simulink model "Dynamics_v2_temp"  (R2021b)
settings: Solver=VariableStepAuto  StartTime=0.0  StopTime=10.0  RelTol=1e-3
InitFcn:
  | % ************** Initiate forces
  | % f0=[0;0;0;0;0;0];
  | % f0=[0;0;0;0;0;0;0];
  | f_0=[0;0;0];
  | f_m=[0;0];
  | f_e=[0;0;0;0;0;0];
  | % ************** Initiate states
  | q_m=[0;0];
  | q_dot_m=[0;0];
  | P=[0;0;0];
  | V_I0=[0;0;0];
  | % ************** Load main
  | %run(Main.m)
values from neighbouring files (symbols this model uses):
  diag_M = diagonalize(M_frak0, M_frak)    [Create_Robot.m]    (also in Main.m; diagonalize.m = zeros(6*(n+1),6*(n+1)); test_C_Main.m)
  iota0 = [1 0 0; 0 1 0;zeros(3,3);0 0 1]    [Create_Robot.m]    (also in Main.m = eye(6,6); test_C_Main.m)
  M_curly = zeros(n,6,6)    [M_curly.m]
  mu = zeros(6,1)'    [Create_Robot.m]    (also in Main.m; test_C_Main.m)
  Xi_m_matrix = zeros(6*n,n)    [Create_Robot.m]    (also in Main.m; test_C_Main.m)
undefined symbols (not defined in the file or in its folder): Ad_gm_inv, g_bar, M_curly0, Xi_m
(part 1 of 2)
settings Model: Creator=Bmmog  LastModifiedBy=Bmmog

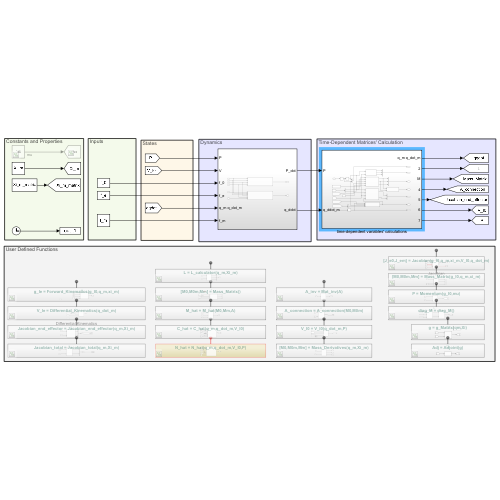
[thumbnail: Simulink's stored preview of the top-level diagram]
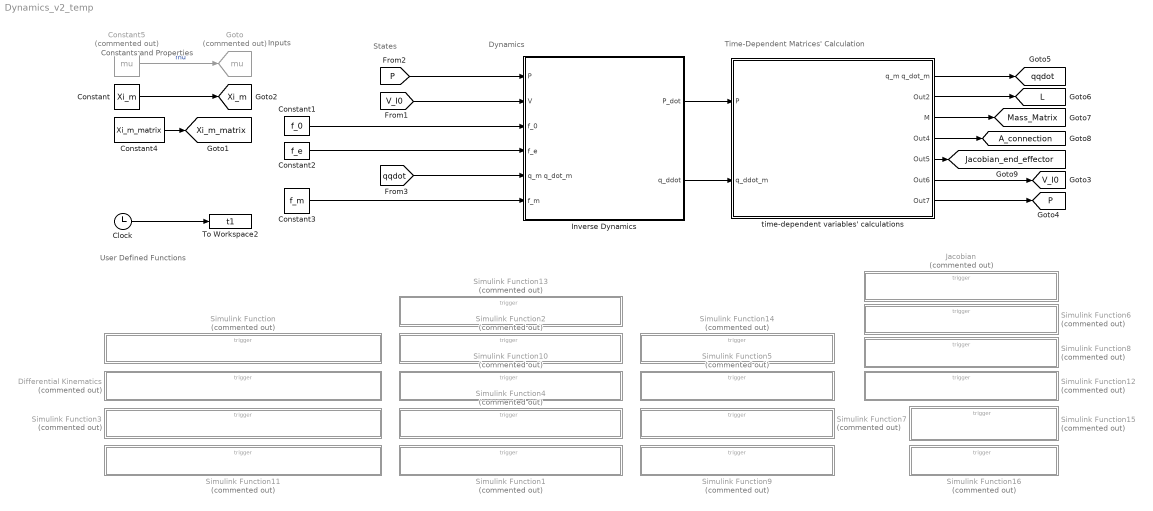
== system Dynamics_v2_temp ==
  note: Time-Dependent Matrices' Calculation
  note: States
  note: Inputs
  note: User Defined Functions
  note: Dynamics
  note: Constants and Properties
  Clock : Clock
  Constant : Constant  Value=Xi_m  VectorParams1D=off
  Constant1 : Constant  Value=f_0  VectorParams1D=off
  Constant2 : Constant  Value=f_e  VectorParams1D=off
  Constant3 : Constant  Value=f_m  VectorParams1D=off
  Constant4 : Constant  Value=Xi_m_matrix  VectorParams1D=off
  Constant5 : Constant  Commented=on  Value=mu
  Differential Kinematics : Subsystem  Commented=on  TreatAsAtomicUnit=on
  Goto : Goto  Commented=on  GotoTag=mu  TagVisibility=global
  Inverse Dynamics : Subsystem
  Jacobian : Subsystem  Commented=on  TreatAsAtomicUnit=on
  Simulink Function : Subsystem  Commented=on  TreatAsAtomicUnit=on
  Simulink Function1 : Subsystem  Commented=on  TreatAsAtomicUnit=on
  Simulink Function10 : Subsystem  Commented=on  TreatAsAtomicUnit=on
  Simulink Function11 : Subsystem  Commented=on  TreatAsAtomicUnit=on
  Simulink Function12 : Subsystem  Commented=on  TreatAsAtomicUnit=on
  Simulink Function13 : Subsystem  Commented=on  TreatAsAtomicUnit=on
  Simulink Function14 : Subsystem  Commented=on  TreatAsAtomicUnit=on
  Simulink Function15 : Subsystem  Commented=on  TreatAsAtomicUnit=on
  Simulink Function16 : Subsystem  Commented=on  TreatAsAtomicUnit=on
  Simulink Function2 : Subsystem  Commented=on  TreatAsAtomicUnit=on
  Simulink Function3 : Subsystem  Commented=on  TreatAsAtomicUnit=on
  Simulink Function4 : Subsystem  Commented=on  TreatAsAtomicUnit=on
  Simulink Function5 : Subsystem  Commented=on  TreatAsAtomicUnit=on
  Simulink Function6 : Subsystem  Commented=on  TreatAsAtomicUnit=on
  Simulink Function7 : Subsystem  Commented=on  TreatAsAtomicUnit=on
  Simulink Function8 : Subsystem  Commented=on  TreatAsAtomicUnit=on
  Simulink Function9 : Subsystem  Commented=on  TreatAsAtomicUnit=on
  To Workspace2 : ToWorkspace  VariableName=t1  SampleTime=-1
  time-dependent variables' calculations : Subsystem
  tag scope: A_connection=global, Jacobian_end_effector=global, L=global, Mass_Matrix=global, P=global, V_I0=global, Xi_m=global, Xi_m_matrix=global, qqdot=global
  wires:
  Constant5/1 -> Goto/1  "mu"
  Clock/1 -> To Workspace2/1
  Constant/1 -> [Xi_m]
  Constant4/1 -> [Xi_m_matrix]
  Constant1/1 -> Inverse Dynamics/3(f_0)
  Constant2/1 -> Inverse Dynamics/4(f_e)
  Constant3/1 -> Inverse Dynamics/6(f_m)
  [P] -> Inverse Dynamics/1(P)
  [V_I0] -> Inverse Dynamics/2(V)
  [qqdot] -> Inverse Dynamics/5(q_m q_dot_m)
  time-dependent variables' calculations/7(Out7) -> [P]
  time-dependent variables' calculations/6(Out6) -> [V_I0]
  time-dependent variables' calculations/5(Out5) -> [Jacobian_end_effector]
  time-dependent variables' calculations/4(Out4) -> [A_connection]
  time-dependent variables' calculations/3(M) -> [Mass_Matrix]
  time-dependent variables' calculations/2(Out2) -> [L]
  time-dependent variables' calculations/1(q_m q_dot_m) -> [qqdot]
  Inverse Dynamics/1(P_dot) -> time-dependent variables' calculations/1(P)
  Inverse Dynamics/2(q_ddot) -> time-dependent variables' calculations/2(q_ddot_m)

== system Dynamics_v2_temp/Differential Kinematics ==
  Differential_Kinematics : TriggerPort  TriggerType=function-call  IsSimulinkFunction=on  FunctionName=Differential_Kinematics  FunctionVisibility=scoped  VariantControl=(inherit)
  Demux : Demux  Outputs=2
  From2 : From  Commented=on  GotoTag=A_connection  TagVisibility=global
  MATLAB Function : MATLAB Function  TreatAsAtomicUnit=on
  q_dot_m : ArgIn  DisableCoverage=on  ArgumentName=q_dot_m
  V_Ie : ArgOut  DisableCoverage=on  ArgumentName=V_Ie
  wires:
  MATLAB Function/1(V_Ie) -> V_Ie/1
  q_dot_m/1 -> MATLAB Function/1(q_dot_m)
  Demux/1 -> MATLAB Function/2(J_e0)
  Demux/2 -> MATLAB Function/3(J_em)
  [Jacobian_end_effector] -> Demux/1
  [V_I0] -> MATLAB Function/4(V_I0)

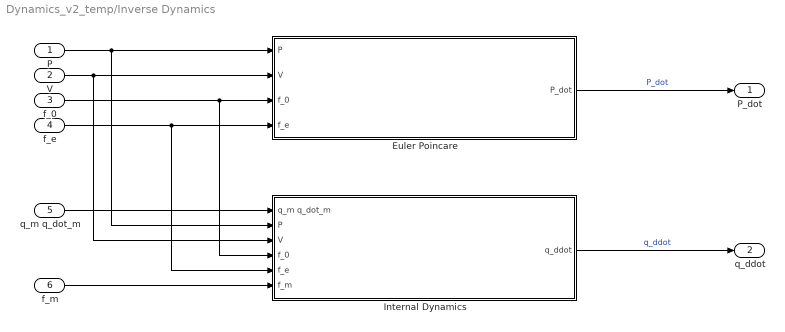
== system Dynamics_v2_temp/Inverse Dynamics ==
  P : Inport
  V : Inport  Port=2
  f_0 : Inport  Port=3
  f_e : Inport  Port=4
  q_m q_dot_m : Inport  Port=5
  f_m : Inport  Port=6
  Euler Poincare : Subsystem
  Internal Dynamics : Subsystem
  P_dot : Outport
  q_ddot : Outport  Port=2
  wires:
  f_0/1 -> Internal Dynamics/4(f_0), Euler Poincare/3(f_0)
  f_e/1 -> Internal Dynamics/5(f_e), Euler Poincare/4(f_e)
  f_m/1 -> Internal Dynamics/6(f_m)
  Internal Dynamics/1(q_ddot) -> q_ddot/1  "q_ddot"
  Euler Poincare/1(P_dot) -> P_dot/1  "P_dot"
  q_m q_dot_m/1 -> Internal Dynamics/1(q_m q_dot_m)
  P/1 -> Internal Dynamics/2(P), Euler Poincare/1(P)
  V/1 -> Internal Dynamics/3(V), Euler Poincare/2(V)

== system Dynamics_v2_temp/Jacobian ==
  Jacobian : TriggerPort  TriggerType=function-call  IsSimulinkFunction=on  FunctionName=Jacobian  FunctionVisibility=scoped  VariantControl=(inherit)
  MATLAB Function : MATLAB Function  TreatAsAtomicUnit=on
  g_I0 : ArgIn  DisableCoverage=on  ArgumentName=g_I0
  q_m : ArgIn  DisableCoverage=on  Port=2  ArgumentName=q_m
  xi_m : ArgIn  DisableCoverage=on  Port=3  ArgumentName=xi_m
  V_I0 : ArgIn  DisableCoverage=on  Port=4  ArgumentName=V_I0
  q_dot_m : ArgIn  DisableCoverage=on  Port=5  ArgumentName=q_dot_m
  J_e0 : ArgOut  DisableCoverage=on  ArgumentName=J_e0
  J_em : ArgOut  DisableCoverage=on  Port=2  ArgumentName=J_em
  wires:
  g_I0/1 -> MATLAB Function/1(robot)
  MATLAB Function/1(J) -> J_e0/1
  q_m/1 -> MATLAB Function/2(q)
  xi_m/1 -> ?
  q_dot_m/1 -> ?
  V_I0/1 -> ?
  ? -> J_em/1

== system Dynamics_v2_temp/Simulink Function ==
  Forward_Kinematics : TriggerPort  TriggerType=function-call  IsSimulinkFunction=on  FunctionName=Forward_Kinematics  FunctionVisibility=scoped  VariantControl=(inherit)
  Constant : Constant  Value=g_bar
  From : From  Commented=on  GotoTag=g_bar
  MATLAB Function : MATLAB Function  TreatAsAtomicUnit=on
  g_I0 : ArgIn  DisableCoverage=on  ArgumentName=g_I0
  q_m : ArgIn  DisableCoverage=on  Port=2  ArgumentName=q_m
  xi_m : ArgIn  DisableCoverage=on  Port=3  ArgumentName=xi_m
  g_Ie : ArgOut  DisableCoverage=on  ArgumentName=g_Ie
  wires:
  g_I0/1 -> MATLAB Function/1(g_I0)
  MATLAB Function/1(g_Ie) -> g_Ie/1
  q_m/1 -> MATLAB Function/2(q_m)
  xi_m/1 -> MATLAB Function/3(Xi_m)
  Constant/1 -> MATLAB Function/4(g_bar)

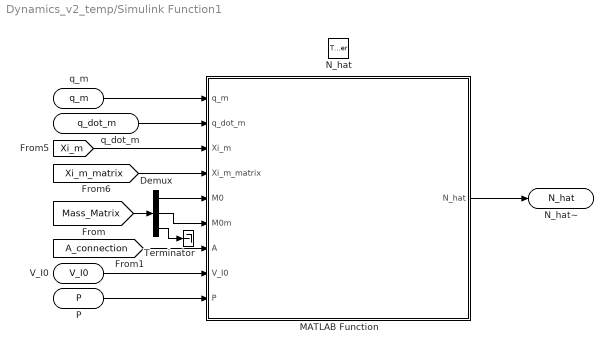
== system Dynamics_v2_temp/Simulink Function1 ==
  N_hat : TriggerPort  TriggerType=function-call  IsSimulinkFunction=on  FunctionName=N_hat  FunctionVisibility=scoped  VariantControl=(inherit)
  Demux : Demux  Outputs=3
  MATLAB Function : MATLAB Function  TreatAsAtomicUnit=on
  Terminator : Terminator
  q_m : ArgIn  DisableCoverage=on  ArgumentName=q_m
  q_dot_m : ArgIn  DisableCoverage=on  Port=2  ArgumentName=q_dot_m
  V_I0 : ArgIn  DisableCoverage=on  Port=3  ArgumentName=V_I0
  P : ArgIn  DisableCoverage=on  Port=4  ArgumentName=P
  N_hat~ : ArgOut  DisableCoverage=on  ArgumentName=N_hat
  wires:
  MATLAB Function/1(N_hat) -> N_hat~/1
  q_m/1 -> MATLAB Function/1(q_m)
  [Xi_m] -> MATLAB Function/3(Xi_m)
  q_dot_m/1 -> MATLAB Function/2(q_dot_m)
  [Xi_m_matrix] -> MATLAB Function/4(Xi_m_matrix)
  [Mass_Matrix] -> Demux/1
  Demux/1 -> MATLAB Function/5(M0)
  Demux/2 -> MATLAB Function/6(M0m)
  Demux/3 -> Terminator/1
  [A_connection] -> MATLAB Function/7(A)
  V_I0/1 -> MATLAB Function/8(V_I0)
  P/1 -> MATLAB Function/9(P)

== system Dynamics_v2_temp/Simulink Function10 ==
  M_hat : TriggerPort  TriggerType=function-call  IsSimulinkFunction=on  FunctionName=M_hat  FunctionVisibility=scoped  VariantControl=(inherit)
  MATLAB Function : MATLAB Function  TreatAsAtomicUnit=on
  M0 : ArgIn  DisableCoverage=on  ArgumentName=M0
  M0m : ArgIn  DisableCoverage=on  Port=2  ArgumentName=Mm
  A : ArgIn  DisableCoverage=on  Port=3  ArgumentName=A
  M_hat~ : ArgOut  DisableCoverage=on  ArgumentName=M_hat
  wires:
  MATLAB Function/1(M_hat) -> M_hat~/1
  M0m/1 -> MATLAB Function/2(Mm)
  A/1 -> MATLAB Function/3(A)
  M0/1 -> MATLAB Function/1(M0)

== system Dynamics_v2_temp/Simulink Function11 ==
  Jacobian_total : TriggerPort  TriggerType=function-call  IsSimulinkFunction=on  FunctionName=Jacobian_total  FunctionVisibility=scoped  VariantControl=(inherit)
  MATLAB Function : MATLAB Function  TreatAsAtomicUnit=on
  Mux : Mux  Inputs=2
  q_m : ArgIn  DisableCoverage=on  ArgumentName=q_m
  Xi_m : ArgIn  DisableCoverage=on  Port=2  ArgumentName=Xi_m
  Jacobian_total~ : ArgOut  DisableCoverage=on  ArgumentName=Jacobian_total
  wires:
  MATLAB Function/1(J_e0) -> Mux/1
  q_m/1 -> MATLAB Function/1(q_m)
  Xi_m/1 -> MATLAB Function/2(Xi_m)
  MATLAB Function/2(J_em) -> Mux/2
  Mux/1 -> Jacobian_total~/1

== system Dynamics_v2_temp/Simulink Function12 ==
  diag_M : TriggerPort  TriggerType=function-call  IsSimulinkFunction=on  FunctionName=diag_M  FunctionVisibility=scoped  VariantControl=(inherit)
  Constant : Constant  Value=M_curly0
  Constant1 : Constant  Value=M_curly
  Constant2 : Constant  Value=Ad_gm_inv
  MATLAB Function : MATLAB Function  TreatAsAtomicUnit=on
  MATLAB Function1 : MATLAB Function  TreatAsAtomicUnit=on
  diag_M~ : ArgOut  DisableCoverage=on  ArgumentName=diag_M
  wires:
  MATLAB Function/2(M_frak) -> MATLAB Function1/2(M_frak)
  MATLAB Function1/1(diag_M) -> diag_M~/1
  Constant/1 -> MATLAB Function/1(M_curly0)
  Constant1/1 -> MATLAB Function/2(M_curly)
  Constant2/1 -> MATLAB Function/3(Ad_gm_inv)
  MATLAB Function/1(M_frak0) -> MATLAB Function1/1(M_frak0)

== system Dynamics_v2_temp/Simulink Function13 ==
  L_calculator : TriggerPort  TriggerType=function-call  IsSimulinkFunction=on  FunctionName=L_calculator  FunctionVisibility=scoped  VariantControl=(inherit)
  " " : MATLAB Function  TreatAsAtomicUnit=on
  Mux : Mux  Inputs=3
  q_m : ArgIn  DisableCoverage=on  ArgumentName=q_m
  Xi_m : ArgIn  DisableCoverage=on  Port=2  ArgumentName=Xi_m
  L : ArgOut  DisableCoverage=on  ArgumentName=L
  wires:
  " "/1(L0) -> Mux/1
  Xi_m/1 -> " "/2(Xi_m)
  " "/2(Lm0) -> Mux/2
  Mux/1 -> L/1
  " "/3(Lm) -> Mux/3
  q_m/1 -> " "/1(q_m)

== system Dynamics_v2_temp/Simulink Function14 ==
  Mat_inv : TriggerPort  TriggerType=function-call  IsSimulinkFunction=on  FunctionName=Mat_inv  FunctionVisibility=scoped  VariantControl=(inherit)
  MATLAB Function1 : MATLAB Function  TreatAsAtomicUnit=on
  A : ArgIn  DisableCoverage=on  ArgumentName=A
  A_inv : ArgOut  DisableCoverage=on  ArgumentName=A_inv
  wires:
  A/1 -> MATLAB Function1/1(A)
  MATLAB Function1/1(A_inv) -> A_inv/1

== system Dynamics_v2_temp/Simulink Function15 ==
  g_Matrix : TriggerPort  TriggerType=function-call  IsSimulinkFunction=on  FunctionName=g_Matrix  FunctionVisibility=scoped  VariantControl=(inherit)
  MATLAB Function : MATLAB Function  Commented=on  TreatAsAtomicUnit=on
  MATLAB Function1 : MATLAB Function  TreatAsAtomicUnit=on
  qm : ArgIn  DisableCoverage=on  ArgumentName=qm
  Xi : ArgIn  DisableCoverage=on  Port=2  ArgumentName=Xi
  g : ArgOut  DisableCoverage=on  ArgumentName=g
  wires:
  qm/1 -> MATLAB Function1/2(qm)
  Xi/1 -> MATLAB Function1/1(xi)
  MATLAB Function1/1(g) -> g/1

== system Dynamics_v2_temp/Simulink Function16 ==
  Adjoint : TriggerPort  TriggerType=function-call  IsSimulinkFunction=on  FunctionName=Adjoint  FunctionVisibility=scoped  VariantControl=(inherit)
  MATLAB Function : MATLAB Function  TreatAsAtomicUnit=on
  u : ArgIn  DisableCoverage=on  ArgumentName=g
  y : ArgOut  DisableCoverage=on  ArgumentName=Adj
  wires:
  u/1 -> MATLAB Function/1(g)
  MATLAB Function/1(Adj) -> y/1

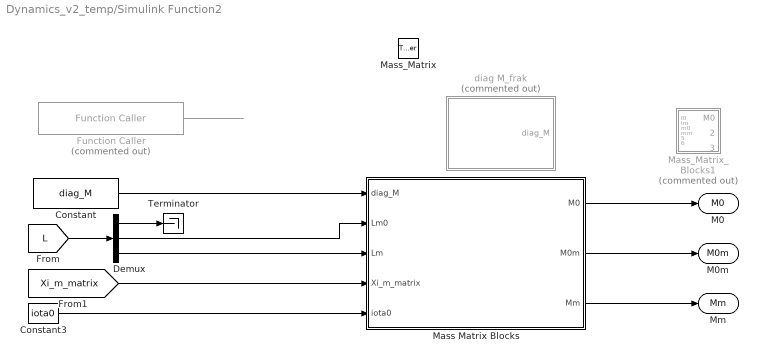
== system Dynamics_v2_temp/Simulink Function2 ==
  Mass_Matrix : TriggerPort  TriggerType=function-call  IsSimulinkFunction=on  FunctionName=Mass_Matrix  FunctionVisibility=scoped  VariantControl=(inherit)
  Constant : Constant  Value=diag_M  VectorParams1D=off
  Constant3 : Constant  Value=iota0  VectorParams1D=off
  Demux : Demux  Outputs=3
  Function Caller : FunctionCaller  Commented=on  FunctionPrototype=diag_M = diag_M()  InputArgumentSpecifications=<Enter example>  OutputArgumentSpecifications=<Enter example>
  Mass Matrix Blocks : Subsystem
  Mass_Matrix_Blocks1 : MATLAB Function  Commented=on  TreatAsAtomicUnit=on
  Terminator : Terminator
  diag M_frak : Subsystem  Commented=on
  M0 : ArgOut  DisableCoverage=on  ArgumentName=M0
  M0m : ArgOut  DisableCoverage=on  Port=2  ArgumentName=M0m
  Mm : ArgOut  DisableCoverage=on  Port=3  ArgumentName=Mm
  wires:
  [L] -> Demux/1
  Demux/1 -> Terminator/1
  Demux/2 -> Mass Matrix Blocks/2(Lm0)
  Demux/3 -> Mass Matrix Blocks/3(Lm)
  [Xi_m_matrix] -> Mass Matrix Blocks/4(Xi_m_matrix)
  Constant3/1 -> Mass Matrix Blocks/5(iota0)
  Mass Matrix Blocks/1(M0) -> M0/1
  Mass Matrix Blocks/2(M0m) -> M0m/1
  Mass Matrix Blocks/3(Mm) -> Mm/1
  Function Caller/1 -> ?
  Constant/1 -> Mass Matrix Blocks/1(diag_M)

== system Dynamics_v2_temp/Simulink Function3 ==
  Jacobian_end_effector : TriggerPort  TriggerType=function-call  IsSimulinkFunction=on  FunctionName=Jacobian_end_effector  FunctionVisibility=scoped  VariantControl=(inherit)
  MATLAB Function : MATLAB Function  TreatAsAtomicUnit=on
  Mux : Mux  Inputs=2
  q_m : ArgIn  DisableCoverage=on  ArgumentName=q_m
  Xi_m : ArgIn  DisableCoverage=on  Port=2  ArgumentName=Xi_m
  Jacobian_end_effector~ : ArgOut  DisableCoverage=on  ArgumentName=Jacobian_end_effector
  wires:
  MATLAB Function/1(J_e0) -> Mux/1
  q_m/1 -> MATLAB Function/1(q_m)
  Xi_m/1 -> MATLAB Function/2(Xi_m)
  MATLAB Function/2(J_em) -> Mux/2
  Mux/1 -> Jacobian_end_effector~/1

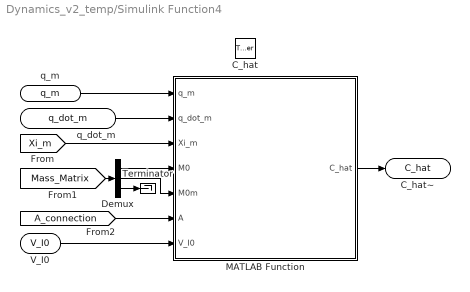
== system Dynamics_v2_temp/Simulink Function4 ==
  C_hat : TriggerPort  TriggerType=function-call  IsSimulinkFunction=on  FunctionName=C_hat  FunctionVisibility=scoped  VariantControl=(inherit)
  Demux : Demux  Outputs=3
  MATLAB Function : MATLAB Function  TreatAsAtomicUnit=on
  Terminator : Terminator
  q_m : ArgIn  DisableCoverage=on  ArgumentName=q_m
  q_dot_m : ArgIn  DisableCoverage=on  Port=2  ArgumentName=q_dot_m
  V_I0 : ArgIn  DisableCoverage=on  Port=3  ArgumentName=V_I0
  C_hat~ : ArgOut  DisableCoverage=on  ArgumentName=C_hat
  wires:
  [Mass_Matrix] -> Demux/1
  MATLAB Function/1(C_hat) -> C_hat~/1
  q_m/1 -> MATLAB Function/1(q_m)
  [Xi_m] -> MATLAB Function/3(Xi_m)
  q_dot_m/1 -> MATLAB Function/2(q_dot_m)
  [A_connection] -> MATLAB Function/6(A)
  Demux/3 -> Terminator/1
  Demux/1 -> MATLAB Function/4(M0)
  Demux/2 -> MATLAB Function/5(M0m)
  V_I0/1 -> MATLAB Function/7(V_I0)

== system Dynamics_v2_temp/Simulink Function5 ==
  A_connection : TriggerPort  TriggerType=function-call  IsSimulinkFunction=on  FunctionName=A_connection  FunctionVisibility=scoped  VariantControl=(inherit)
  MATLAB Function : MATLAB Function  TreatAsAtomicUnit=on
  M0 : ArgIn  DisableCoverage=on  ArgumentName=M0
  M0m : ArgIn  DisableCoverage=on  Port=2  ArgumentName=M0m
  A_connection~ : ArgOut  DisableCoverage=on  ArgumentName=A_connection
  wires:
  M0/1 -> MATLAB Function/1(M0)
  MATLAB Function/1(A) -> A_connection~/1
  M0m/1 -> MATLAB Function/2(M0m)

== system Dynamics_v2_temp/Simulink Function6 ==
  Mass_Matrix : TriggerPort  TriggerType=function-call  IsSimulinkFunction=on  FunctionName=Mass_Matrix  FunctionVisibility=scoped  VariantControl=(inherit)
  MATLAB Function : MATLAB Function  TreatAsAtomicUnit=on
  g_I0 : ArgIn  DisableCoverage=on  ArgumentName=g_I0
  q_m : ArgIn  DisableCoverage=on  Port=2  ArgumentName=q_m
  xi_m : ArgIn  DisableCoverage=on  Port=3  ArgumentName=xi_m
  M0 : ArgOut  DisableCoverage=on  ArgumentName=M0
  M0m : ArgOut  DisableCoverage=on  Port=2  ArgumentName=M0m
  Mm : ArgOut  DisableCoverage=on  Port=3  ArgumentName=Mm
  wires:
  g_I0/1 -> MATLAB Function/1(I0)
  MATLAB Function/1(M0) -> M0/1
  q_m/1 -> MATLAB Function/7(q_m)
  xi_m/1 -> MATLAB Function/8(Xi_m)
  MATLAB Function/2(M0m) -> M0m/1
  MATLAB Function/3(Mm) -> Mm/1

== system Dynamics_v2_temp/Simulink Function7 ==
  V_I0 : TriggerPort  TriggerType=function-call  IsSimulinkFunction=on  FunctionName=V_I0  FunctionVisibility=scoped  VariantControl=(inherit)
  Demux : Demux  Outputs=3
  MATLAB Function : MATLAB Function  TreatAsAtomicUnit=on
  Terminator : Terminator
  Terminator1 : Terminator
  q_dot_m : ArgIn  DisableCoverage=on  ArgumentName=q_dot_m
  P : ArgIn  DisableCoverage=on  Port=2  ArgumentName=P
  V_I0~ : ArgOut  DisableCoverage=on  ArgumentName=V_I0
  wires:
  Demux/1 -> MATLAB Function/4(M0)
  MATLAB Function/1(V_I0) -> V_I0~/1
  P/1 -> MATLAB Function/1(P)
  [Mass_Matrix] -> Demux/1
  Demux/2 -> Terminator/1
  Demux/3 -> Terminator1/1
  [A_connection] -> MATLAB Function/2(A_connection)
  q_dot_m/1 -> MATLAB Function/3(q_dot_m)

== system Dynamics_v2_temp/Simulink Function8 ==
  Momentum : TriggerPort  TriggerType=function-call  IsSimulinkFunction=on  FunctionName=Momentum  FunctionVisibility=scoped  VariantControl=(inherit)
  MATLAB Function : MATLAB Function  TreatAsAtomicUnit=on
  g_I0 : ArgIn  DisableCoverage=on  ArgumentName=g_I0
  mu : ArgIn  DisableCoverage=on  Port=2  ArgumentName=mu
  P : ArgOut  DisableCoverage=on  ArgumentName=P
  wires:
  MATLAB Function/1(P) -> P/1
  g_I0/1 -> MATLAB Function/1(g_I0)
  mu/1 -> MATLAB Function/2(mu)

== system Dynamics_v2_temp/Simulink Function9 ==
  Mass_Derivatives : TriggerPort  TriggerType=function-call  IsSimulinkFunction=on  FunctionName=Mass_Derivatives  FunctionVisibility=scoped  VariantControl=(inherit)
  MATLAB Function : MATLAB Function  TreatAsAtomicUnit=on
  q_m : ArgIn  DisableCoverage=on  ArgumentName=q_m
  xi_m : ArgIn  DisableCoverage=on  Port=2  ArgumentName=Xi_m
  M0 : ArgOut  DisableCoverage=on  ArgumentName=M0
  M0m : ArgOut  DisableCoverage=on  Port=2  ArgumentName=M0m
  Mm : ArgOut  DisableCoverage=on  Port=3  ArgumentName=Mm
  wires:
  MATLAB Function/1(M0_partial) -> M0/1
  q_m/1 -> MATLAB Function/1(q_m)
  xi_m/1 -> MATLAB Function/2(Xi_m)
  MATLAB Function/2(M0m_partial) -> M0m/1
  MATLAB Function/3(Mm_partial) -> Mm/1

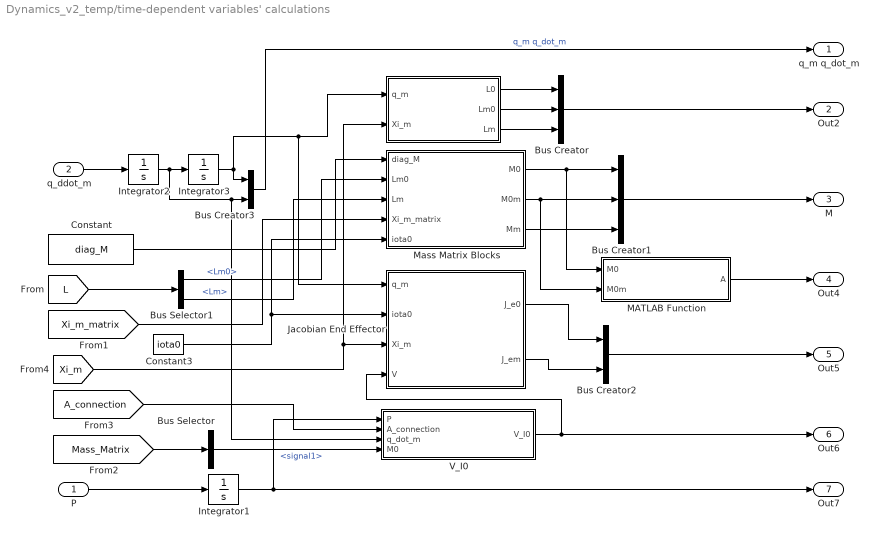
== system Dynamics_v2_temp/time-dependent variables' calculations ==
  P : Inport
  q_ddot_m : Inport  Port=2
  " " : MATLAB Function  TreatAsAtomicUnit=on
  Bus Creator : BusCreator  Inputs=3
  Bus Creator1 : BusCreator  Inputs=3
  Bus Creator2 : BusCreator  Inputs=2
  Bus Creator3 : BusCreator  Inputs=2
  Bus Selector : BusSelector  OutputSignals=signal1
  Bus Selector1 : BusSelector  OutputSignals=Lm0,Lm
  Constant : Constant  Value=diag_M  VectorParams1D=off
  Constant3 : Constant  Value=iota0  VectorParams1D=off
  Integrator1 : Integrator
  Integrator2 : Integrator
  Integrator3 : Integrator
  Jacobian End Effector : Subsystem
  MATLAB Function : MATLAB Function  TreatAsAtomicUnit=on
  Mass Matrix Blocks : Subsystem
  V_I0 : MATLAB Function  TreatAsAtomicUnit=on
  q_m q_dot_m : Outport
  Out2 : Outport  Port=2
  M : Outport  Port=3
  Out4 : Outport  Port=4
  Out5 : Outport  Port=5
  Out6 : Outport  Port=6
  Out7 : Outport  Port=7
  wires:
  Mass Matrix Blocks/3(Mm) -> Bus Creator1/3
  Mass Matrix Blocks/2(M0m) -> MATLAB Function/2(M0m), Bus Creator1/2
  Integrator2/1 -> V_I0/3(q_dot_m), Bus Creator3/2, Integrator3/1
  Bus Creator3/1 -> q_m q_dot_m/1  "q_m q_dot_m"
  Mass Matrix Blocks/1(M0) -> MATLAB Function/1(M0), Bus Creator1/1
  Integrator1/1 -> Out7/1, V_I0/1(P)
  q_ddot_m/1 -> Integrator2/1
  V_I0/1(V_I0) -> Jacobian End Effector/4(V), Out6/1
  Bus Creator2/1 -> Out5/1
  MATLAB Function/1(A) -> Out4/1
  Bus Creator1/1 -> M/1
  P/1 -> Integrator1/1
  " "/1(L0) -> Bus Creator/1
  " "/3(Lm) -> Bus Creator/3
  " "/2(Lm0) -> Bus Creator/2
  Bus Creator/1 -> Out2/1
  Constant3/1 -> Mass Matrix Blocks/5(iota0), Jacobian End Effector/2(iota0)
  Constant/1 -> Mass Matrix Blocks/1(diag_M)
  Bus Selector1/2 -> Mass Matrix Blocks/3(Lm)  "<Lm>"
  [Xi_m_matrix] -> Mass Matrix Blocks/4(Xi_m_matrix)
  Bus Selector1/1 -> Mass Matrix Blocks/2(Lm0)  "<Lm0>"
  [L] -> Bus Selector1/1
  [A_connection] -> V_I0/2(A_connection)
  Bus Selector/1 -> V_I0/4(M0)  "<signal1>"
  [Mass_Matrix] -> Bus Selector/1
  [Xi_m] -> " "/2(Xi_m), Jacobian End Effector/3(Xi_m)
  Integrator3/1 -> Bus Creator3/1, Jacobian End Effector/1(q_m), " "/1(q_m)
  Jacobian End Effector/1(J_e0) -> Bus Creator2/1
  Jacobian End Effector/2(J_em) -> Bus Creator2/2

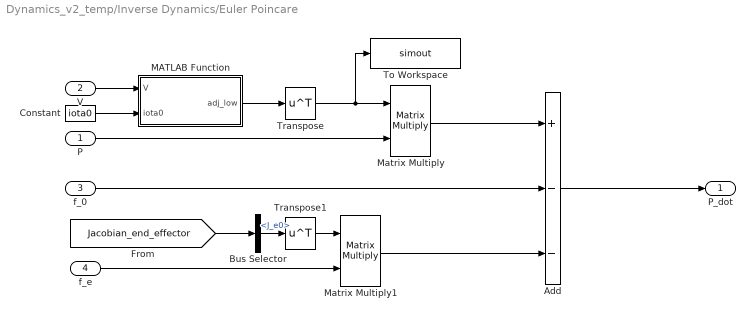
== system Dynamics_v2_temp/Inverse Dynamics/Euler Poincare ==
  P : Inport
  V : Inport  Port=2
  f_0 : Inport  Port=3
  f_e : Inport  Port=4
  Add : Sum  Inputs=+--
  Bus Selector : BusSelector  OutputSignals=J_e0
  Constant : Constant  Value=iota0
  MATLAB Function : MATLAB Function  TreatAsAtomicUnit=on
  Matrix Multiply : Product  Multiplication=Matrix(*)
  Matrix Multiply1 : Product  Multiplication=Matrix(*)
  To Workspace : ToWorkspace  VariableName=simout  SaveFormat=Timeseries  SampleTime=-1
  Transpose : Math  Operator=transpose  SaturateOnIntegerOverflow=on
  Transpose1 : Math  Operator=transpose  SaturateOnIntegerOverflow=on
  P_dot : Outport
  wires:
  P/1 -> Matrix Multiply/2
  MATLAB Function/1(adj_low) -> Transpose/1
  V/1 -> MATLAB Function/1(V)
  Transpose/1 -> To Workspace/1, Matrix Multiply/1
  Matrix Multiply/1 -> Add/1
  f_0/1 -> Add/2
  Add/1 -> P_dot/1
  [Jacobian_end_effector] -> Bus Selector/1
  Bus Selector/1 -> Transpose1/1  "<J_e0>"
  f_e/1 -> Matrix Multiply1/2
  Matrix Multiply1/1 -> Add/3
  Transpose1/1 -> Matrix Multiply1/1
  Constant/1 -> MATLAB Function/2(iota0)

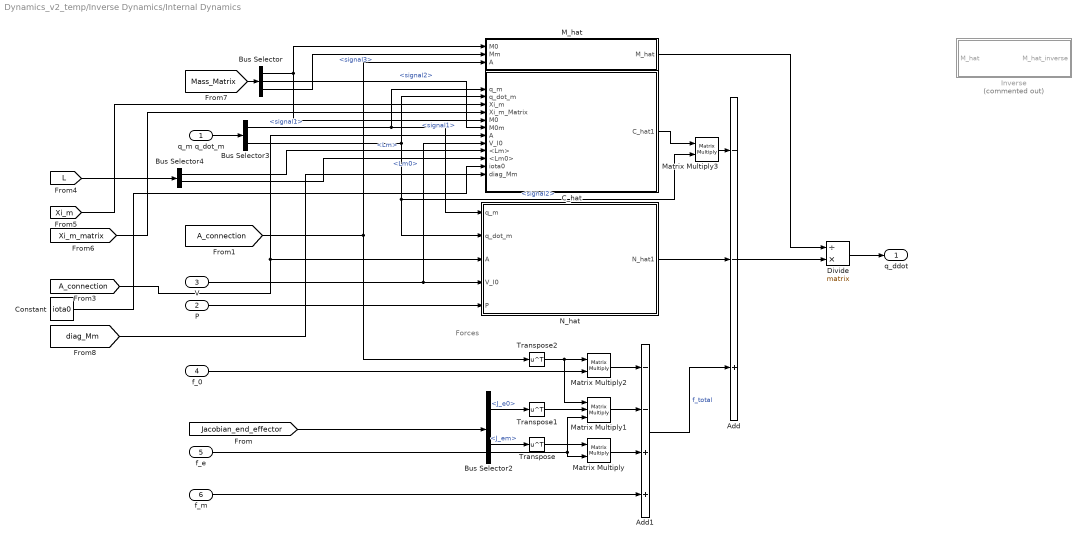
== system Dynamics_v2_temp/Inverse Dynamics/Internal Dynamics ==
  note: Forces
  q_m q_dot_m : Inport
  P : Inport  Port=2
  V : Inport  Port=3
  f_0 : Inport  Port=4
  f_e : Inport  Port=5
  f_m : Inport  Port=6
  Add : Sum  Inputs=--+
  Add1 : Sum  Inputs=--++
  Bus Selector : BusSelector  OutputSignals=signal1,signal2,signal3
  Bus Selector2 : BusSelector  OutputSignals=J_e0,J_em
  Bus Selector3 : BusSelector  OutputSignals=signal1,signal2
  Bus Selector4 : BusSelector  OutputSignals=Lm,Lm0
  C_hat : Subsystem
  Constant : Constant  Value=iota0
  Divide : Product  Inputs=/*  Multiplication=Matrix(*)
  Inverse : MATLAB Function  Commented=on  TreatAsAtomicUnit=on
  M_hat : MATLAB Function  TreatAsAtomicUnit=on
  Matrix Multiply : Product  Multiplication=Matrix(*)
  Matrix Multiply1 : Product  Inputs=3  Multiplication=Matrix(*)
  Matrix Multiply2 : Product  Multiplication=Matrix(*)
  Matrix Multiply3 : Product  Multiplication=Matrix(*)
  N_hat : Subsystem
  Transpose : Math  Operator=transpose  SaturateOnIntegerOverflow=on
  Transpose1 : Math  Operator=transpose  SaturateOnIntegerOverflow=on
  Transpose2 : Math  Operator=transpose  SaturateOnIntegerOverflow=on
  q_ddot : Outport
  wires:
  q_m q_dot_m/1 -> Bus Selector3/1
  Add/1 -> Divide/2
  Add1/1 -> Add/3  "f_total"
  Matrix Multiply2/1 -> Add1/1
  Transpose/1 -> Matrix Multiply/1
  f_m/1 -> Add1/4
  Transpose1/1 -> Matrix Multiply1/2
  f_e/1 -> Matrix Multiply/2, Matrix Multiply1/3
  Matrix Multiply1/1 -> Add1/2
  Bus Selector2/1 -> Transpose1/1  "<J_e0>"
  Matrix Multiply/1 -> Add1/3
  Transpose2/1 -> Matrix Multiply2/1, Matrix Multiply1/1
  [A_connection] -> M_hat/3(A), Transpose2/1
  f_0/1 -> Matrix Multiply2/2
  [Jacobian_end_effector] -> Bus Selector2/1
  Bus Selector2/2 -> Transpose/1  "<J_em>"
  Bus Selector3/1 -> N_hat/1(q_m), C_hat/1(q_m)  "<signal1>"
  Bus Selector3/2 -> Matrix Multiply3/2, N_hat/2(q_dot_m), C_hat/2(q_dot_m)  "<signal2>"
  Matrix Multiply3/1 -> Add/1
  V/1 -> C_hat/8(V_I0), N_hat/4(V_I0)
  [Mass_Matrix] -> Bus Selector/1
  Bus Selector/1 -> C_hat/5(M0), M_hat/1(M0)  "<signal1>"
  Bus Selector/3 -> M_hat/2(Mm)  "<signal3>"
  M_hat/1(M_hat) -> Divide/1
  [A_connection] -> N_hat/3(A), C_hat/7(A)
  [Xi_m_matrix] -> C_hat/4(Xi_m_Matrix)
  [Xi_m] -> C_hat/3(Xi_m)
  [L] -> Bus Selector4/1
  Bus Selector4/1 -> C_hat/9(<Lm>)  "<Lm>"
  Bus Selector4/2 -> C_hat/10(<Lm0>)  "<Lm0>"
  Bus Selector/2 -> C_hat/6(M0m)  "<signal2>"
  Constant/1 -> C_hat/11(iota0)
  [diag_Mm] -> C_hat/12(diag_Mm)
  C_hat/1(C_hat1) -> Matrix Multiply3/1
  P/1 -> N_hat/5(P)
  N_hat/1(N_hat1) -> Add/2
  Divide/1 -> q_ddot/1

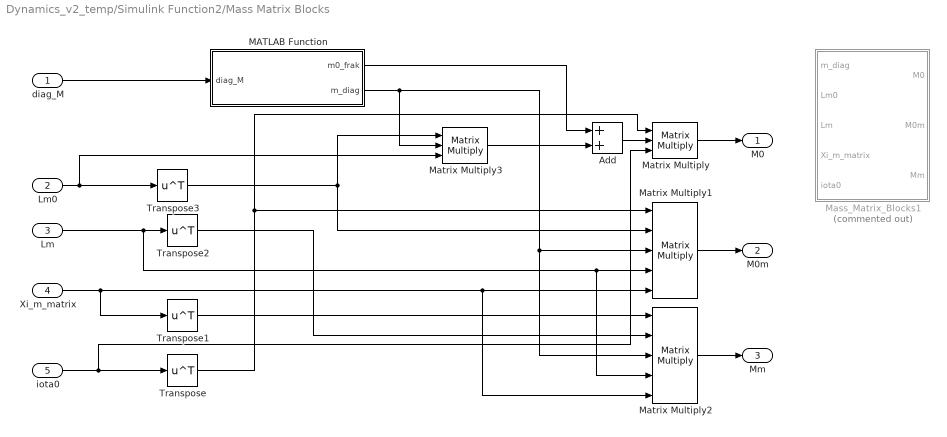
== system Dynamics_v2_temp/Simulink Function2/Mass Matrix Blocks ==
  diag_M : Inport
  Lm0 : Inport  Port=2
  Lm : Inport  Port=3
  Xi_m_matrix : Inport  Port=4
  iota0 : Inport  Port=5
  Add : Sum
  MATLAB Function : MATLAB Function  TreatAsAtomicUnit=on
  Mass_Matrix_Blocks1 : MATLAB Function  Commented=on  TreatAsAtomicUnit=on
  Matrix Multiply : Product  Inputs=3  Multiplication=Matrix(*)
  Matrix Multiply1 : Product  Inputs=5  Multiplication=Matrix(*)
  Matrix Multiply2 : Product  Inputs=5  Multiplication=Matrix(*)
  Matrix Multiply3 : Product  Inputs=3  Multiplication=Matrix(*)
  Transpose{,1..3} (4 alike) : Math  Operator=transpose  SaturateOnIntegerOverflow=on
  M0 : Outport
  M0m : Outport  Port=2
  Mm : Outport  Port=3
  wires:
  Matrix Multiply2/1 -> Mm/1
  Xi_m_matrix/1 -> Transpose1/1, Matrix Multiply1/5, Matrix Multiply2/5
  Lm0/1 -> Matrix Multiply3/3, Transpose3/1
  Matrix Multiply/1 -> M0/1
  diag_M/1 -> MATLAB Function/1(diag_M)
  Matrix Multiply1/1 -> M0m/1
  iota0/1 -> Matrix Multiply/3, Transpose/1
  Lm/1 -> Matrix Multiply1/4, Matrix Multiply2/4, Transpose2/1
  Transpose/1 -> Matrix Multiply/1, Matrix Multiply1/1
  Transpose1/1 -> Matrix Multiply2/1
  Transpose2/1 -> Matrix Multiply2/2
  Transpose3/1 -> Matrix Multiply3/1, Matrix Multiply1/2
  MATLAB Function/2(m_diag) -> Matrix Multiply3/2, Matrix Multiply1/3, Matrix Multiply2/3
  MATLAB Function/1(m0_frak) -> Add/1
  Add/1 -> Matrix Multiply/2
  Matrix Multiply3/1 -> Add/2

== system Dynamics_v2_temp/Simulink Function2/diag M_frak ==
  Function Caller : FunctionCaller  Commented=on  FunctionPrototype=diag_M = diag_M(m0,mm,qm)  InputArgumentSpecifications=<Enter example>  OutputArgumentSpecifications=<Enter example>
  MATLAB Function1 : MATLAB Function  TreatAsAtomicUnit=on
  Subsystem : Subsystem
  diag_M : Outport
  wires:
  MATLAB Function1/1(diag_M) -> diag_M/1
  Subsystem/1(M_frak array1) -> MATLAB Function1/1(M_frak)

== system Dynamics_v2_temp/time-dependent variables' calculations/Jacobian End Effector ==
  q_m : Inport
  iota0 : Inport  Port=2
  Xi_m : Inport  Port=3
  V : Inport  Port=4
  Constant : Constant  Value=g_bar
  Forward Kinematics : MATLAB Function  TreatAsAtomicUnit=on
  Jacobian_ee : MATLAB Function  TreatAsAtomicUnit=on
  J_e0 : Outport
  J_em : Outport  Port=2
  wires:
  Xi_m/1 -> Jacobian_ee/2(Xi_m), Forward Kinematics/2(Xi_m)
  iota0/1 -> Jacobian_ee/4(iota0)
  q_m/1 -> Forward Kinematics/1(q_m), Jacobian_ee/1(q_m)
  Jacobian_ee/1(J_e0) -> J_e0/1
  Forward Kinematics/1(g_0e) -> Jacobian_ee/5(g_0e)
  V/1 -> Jacobian_ee/3(V)
  Jacobian_ee/2(J_em) -> J_em/1
  Constant/1 -> Forward Kinematics/3(g_bar)

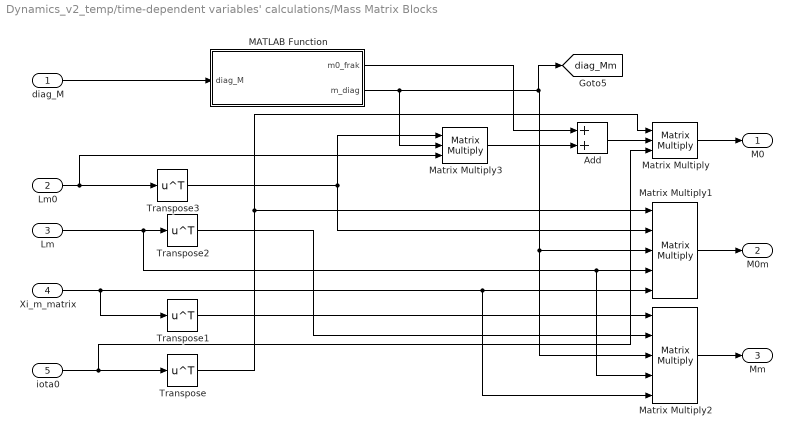
== system Dynamics_v2_temp/time-dependent variables' calculations/Mass Matrix Blocks ==
  diag_M : Inport
  Lm0 : Inport  Port=2
  Lm : Inport  Port=3
  Xi_m_matrix : Inport  Port=4
  iota0 : Inport  Port=5
  Add : Sum
  MATLAB Function : MATLAB Function  TreatAsAtomicUnit=on
  Matrix Multiply : Product  Inputs=3  Multiplication=Matrix(*)
  Matrix Multiply1 : Product  Inputs=5  Multiplication=Matrix(*)
  Matrix Multiply2 : Product  Inputs=5  Multiplication=Matrix(*)
  Matrix Multiply3 : Product  Inputs=3  Multiplication=Matrix(*)
  Transpose{,1..3} (4 alike) : Math  Operator=transpose  SaturateOnIntegerOverflow=on
  M0 : Outport
  M0m : Outport  Port=2
  Mm : Outport  Port=3
  tag scope: diag_Mm=global
  wires:
  Matrix Multiply2/1 -> Mm/1
  Xi_m_matrix/1 -> Transpose1/1, Matrix Multiply1/5, Matrix Multiply2/5
  Lm0/1 -> Matrix Multiply3/3, Transpose3/1
  Matrix Multiply/1 -> M0/1
  diag_M/1 -> MATLAB Function/1(diag_M)
  Matrix Multiply1/1 -> M0m/1
  iota0/1 -> Matrix Multiply/3, Transpose/1
  Lm/1 -> Matrix Multiply1/4, Matrix Multiply2/4, Transpose2/1
  Transpose/1 -> Matrix Multiply/1, Matrix Multiply1/1
  Transpose1/1 -> Matrix Multiply2/1
  Transpose2/1 -> Matrix Multiply2/2
  Transpose3/1 -> Matrix Multiply3/1, Matrix Multiply1/2
  MATLAB Function/2(m_diag) -> Matrix Multiply3/2, [diag_Mm], Matrix Multiply1/3, Matrix Multiply2/3
  MATLAB Function/1(m0_frak) -> Add/1
  Add/1 -> Matrix Multiply/2
  Matrix Multiply3/1 -> Add/2

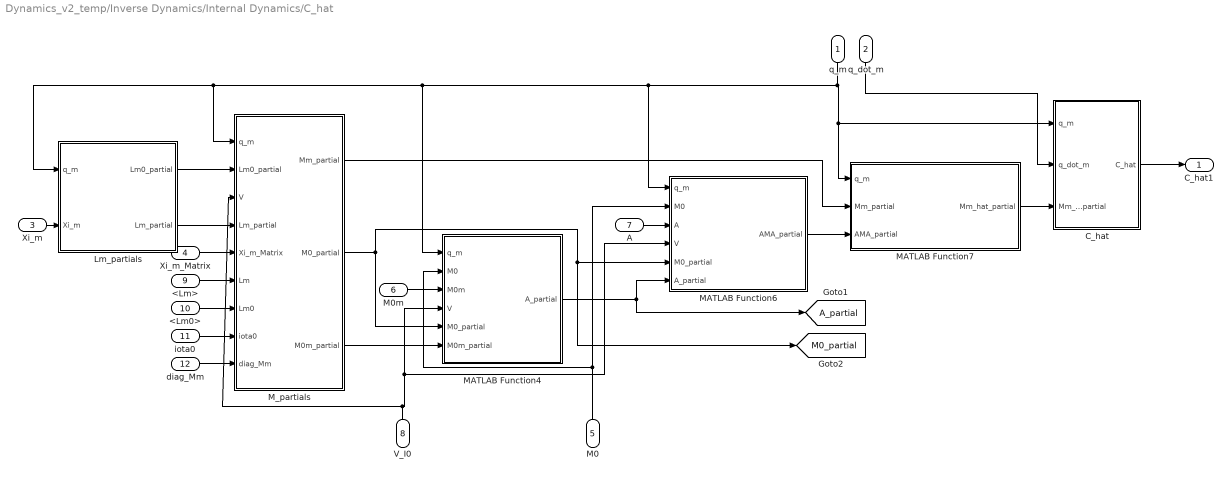
== system Dynamics_v2_temp/Inverse Dynamics/Internal Dynamics/C_hat ==
  q_m : Inport
  q_dot_m : Inport  Port=2
  Xi_m : Inport  Port=3
  Xi_m_Matrix : Inport  Port=4
  M0 : Inport  Port=5
  M0m : Inport  Port=6
  A : Inport  Port=7
  V_I0 : Inport  Port=8
  <Lm> : Inport  Port=9
  <Lm0> : Inport  Port=10
  iota0 : Inport  Port=11
  diag_Mm : Inport  Port=12
  C_hat : MATLAB Function  TreatAsAtomicUnit=on
  Lm_partials : Subsystem
  MATLAB Function4 : MATLAB Function  TreatAsAtomicUnit=on
  MATLAB Function6 : MATLAB Function  TreatAsAtomicUnit=on
  MATLAB Function7 : MATLAB Function  TreatAsAtomicUnit=on
  M_partials : Subsystem
  C_hat1 : Outport
  tag scope: A_partial=global, M0_partial=global
  wires:
  M0/1 -> MATLAB Function6/2(M0), MATLAB Function4/2(M0)
  C_hat/1(C_hat) -> C_hat1/1
  q_m/1 -> C_hat/1(q_m), MATLAB Function7/1(q_m), MATLAB Function4/1(q_m), Lm_partials/1(q_m), M_partials/1(q_m), MATLAB Function6/1(q_m)
  q_dot_m/1 -> C_hat/2(q_dot_m)
  V_I0/1 -> MATLAB Function6/4(V), MATLAB Function4/4(V), M_partials/3(V)
  MATLAB Function4/1(A_partial) -> [A_partial], MATLAB Function6/6(A_partial)
  M0m/1 -> MATLAB Function4/3(M0m)
  A/1 -> MATLAB Function6/3(A)
  MATLAB Function6/1(AMA_partial) -> MATLAB Function7/3(AMA_partial)
  MATLAB Function7/1(Mm_hat_partial) -> C_hat/3(Mm_hat_partial)
  M_partials/2(M0_partial) -> MATLAB Function4/5(M0_partial), [M0_partial], MATLAB Function6/5(M0_partial)
  Xi_m_Matrix/1 -> M_partials/5(Xi_m_Matrix)
  <Lm>/1 -> M_partials/6(Lm)
  <Lm0>/1 -> M_partials/7(Lm0)
  iota0/1 -> M_partials/8(iota0)
  diag_Mm/1 -> M_partials/9(diag_Mm)
  M_partials/1(Mm_partial) -> MATLAB Function7/2(Mm_partial)
  M_partials/3(M0m_partial) -> MATLAB Function4/6(M0m_partial)
  Xi_m/1 -> Lm_partials/2(Xi_m)
  Lm_partials/1(Lm0_partial) -> M_partials/2(Lm0_partial)
  Lm_partials/2(Lm_partial) -> M_partials/4(Lm_partial)

== system Dynamics_v2_temp/Inverse Dynamics/Internal Dynamics/N_hat ==
  q_m : Inport
  q_dot_m : Inport  Port=2
  A : Inport  Port=3
  V_I0 : Inport  Port=4
  P : Inport  Port=5
  Constant : Constant  Value=iota0
  N_hat : MATLAB Function  TreatAsAtomicUnit=on
  N_hat1 : Outport
  wires:
  P/1 -> N_hat/5(P)
  [M0_partial] -> N_hat/6(M0_partial)
  N_hat/1(N_hat) -> N_hat1/1
  q_m/1 -> N_hat/1(q_m)
  q_dot_m/1 -> N_hat/2(q_dot_m)
  V_I0/1 -> N_hat/4(V)
  A/1 -> N_hat/3(A)
  [A_partial] -> N_hat/7(A_partial)
  Constant/1 -> N_hat/8(iota0)

== system Dynamics_v2_temp/Simulink Function2/diag M_frak/Subsystem ==
  m0 : Inport
  mm : Inport  Port=2
  M_frak array : MATLAB Function  TreatAsAtomicUnit=on
  M_frak array1 : Outport
  wires:
  m0/1 -> M_frak array/3(M_curlym)
  M_frak array/1(M_frak) -> M_frak array1/1  "M_frak array"
  mm/1 -> M_frak array/1(M_curly0)
  [A_connection] -> M_frak array/5(g_bar)

== system Dynamics_v2_temp/Inverse Dynamics/Internal Dynamics/C_hat/Lm_partials ==
  q_m : Inport
  Xi_m : Inport  Port=2
  Constant : Constant  Value=iota0
  Lm0partial : MATLAB Function  TreatAsAtomicUnit=on
  Lmpartial : MATLAB Function  TreatAsAtomicUnit=on
  Lm0_partial : Outport
  Lm_partial : Outport  Port=2
  wires:
  Xi_m/1 -> Lmpartial/2(Xi_m), Lm0partial/2(Xi_m)
  q_m/1 -> Lmpartial/1(q_m), Lm0partial/1(q_m)
  Lmpartial/1(Lm_partial) -> Lm_partial/1
  Lm0partial/1(Lm0_partial) -> Lm0_partial/1
  Constant/1 -> Lmpartial/3(iota0), Lm0partial/3(iota0)

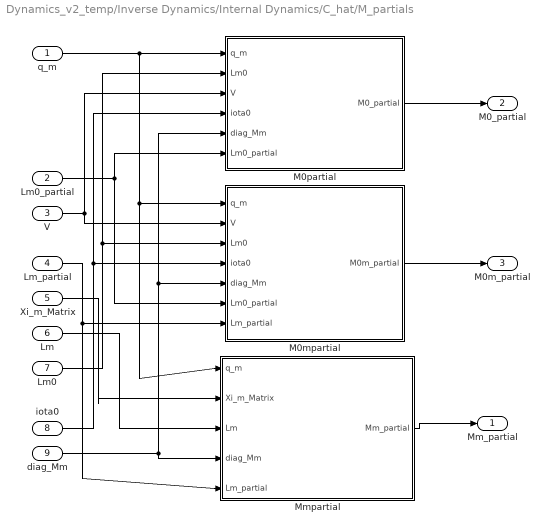
== system Dynamics_v2_temp/Inverse Dynamics/Internal Dynamics/C_hat/M_partials ==
  q_m : Inport
  Lm0_partial : Inport  Port=2
  V : Inport  Port=3
  Lm_partial : Inport  Port=4
  Xi_m_Matrix : Inport  Port=5
  Lm : Inport  Port=6
  Lm0 : Inport  Port=7
  iota0 : Inport  Port=8
  diag_Mm : Inport  Port=9
  " M0partial" : MATLAB Function  TreatAsAtomicUnit=on
  M0mpartial : MATLAB Function  TreatAsAtomicUnit=on
  Mmpartial : MATLAB Function  TreatAsAtomicUnit=on
  Mm_partial : Outport
  M0_partial : Outport  Port=2
  M0m_partial : Outport  Port=3
  wires:
  Lm_partial/1 -> M0mpartial/7(Lm_partial), Mmpartial/5(Lm_partial)
  Lm0_partial/1 -> " M0partial"/6(Lm0_partial), M0mpartial/6(Lm0_partial)
  Lm0/1 -> " M0partial"/2(Lm0), M0mpartial/3(Lm0)
  M0mpartial/1(M0m_partial) -> M0m_partial/1
  q_m/1 -> M0mpartial/1(q_m), Mmpartial/1(q_m), " M0partial"/1(q_m)
  diag_Mm/1 -> M0mpartial/5(diag_Mm), " M0partial"/5(diag_Mm), Mmpartial/4(diag_Mm)
  Xi_m_Matrix/1 -> Mmpartial/2(Xi_m_Matrix)
  iota0/1 -> M0mpartial/4(iota0), " M0partial"/4(iota0)
  Lm/1 -> Mmpartial/3(Lm)
  " M0partial"/1(M0_partial) -> M0_partial/1
  Mmpartial/1(Mm_partial) -> Mm_partial/1
  V/1 -> M0mpartial/2(V), " M0partial"/3(V)

== matlab function Dynamics_v2_temp/Simulink Function3/MATLAB Function ==
  data: J_e0 output; q_m input; Xi_m input; J_em output
function [J_e0, J_em] = Jacobian_end_effector(q_m,Xi_m)
% Calculates the body Velocity of end-effector from base pose and arm joint angles

% Compute the geometric Jacobian of the point rp
%   	rp  point of interest in inertial frame 
%       i   link number

n=length(q_m);

% Initiate
J=zeros(6,6 + n);
% Jm=zeros(6,robot.n);

% Vehicle portion
J0=eye(6,6);
J(1:6,1:6)=J0;

% ____________ Manipulator Jacobian _____________ %

% Initiate
j=1;
Jm=zeros(6,6+n);

Jm(1:6,j)=Xi_m(1:6,j);
for j=2:n %Iterate through all joints
    for i=1:j-1
        temp=Adjoint(g_Matrix(Xi_m(:,i),q_m(i)));
    end
    Jm(1:6,j)=temp*Xi_m(:,j);
end


J_ee0=[J0 Jm(1:6,1:n)];
% J_eeI=Adjoint(g_I0)*J_ee0; % transform to inertia

J_e0=J_ee0(1:6,1:6);
J_em=J_ee0(1:6,7:6+n);

end

== matlab function Dynamics_v2_temp/Simulink Function1/MATLAB Function ==
  data: N_hat output; q_m input; q_dot_m input; Xi_m input; Xi_m_matrix input; M0 input; M0m input; A input; V_I0 input; P input
function N_hat = N_hat(q_m,q_dot_m,Xi_m,Xi_m_matrix, M0,M0m,A,V_I0,P)
% Calculates the N_hat_m matrix from base pose and arm joint angles

n=length(q_m);

V=V_I0;

% Find Lm0
for i=1:n
    Lm0=Ad_frak(1,i,Xi_m,q_m);% equation 63 of TRO
end

% Find partial of Lm0 to joint angles
Lm0_partial=zeros(6*n,6,n); % 6nx6xn
for i=1:n
    for j=1:n
        Lm0_partial(6*(j-1)+1:6*j,1:6,i)=Ad_partial(j,1,i,Xi_m,q_m); % equation 114 of TRO paper
    end
end

% Find partial of M0 to joint angles
M0_partial=zeros(6,6,n); %initiate
for i=1:n
    M0_partial(1:6,1:6,i)= transpose(Lm0_partial(i))*diagM*Lm0+transpose(Lm0)*diagM*Lm0_partial(i); %6x6 %equation 117 of TRO
end

% Find partial of M0m to joint angles
M0m_partial=zeros(6,n,n);
for i=1:n
    M0m_partial(6,n,i)= (transpose(Lm0_partial)*diagM*Lm0+transpose(Lm0)*diagM*Lm)*Xi_m_matrix; % equation 118 of TRO paper
end

% Find partial of connection A to each joint angle
A_partial=zeros(6,n,n);
for i=1:n
    A_partial(6,n,i)=inverse(M0)*M0_partial(1:6,1:6,i)*inverse(M0)*M0m+inverse(M0)*M0m_partial(6,n,i); % Equation 122
end


%Form N_hat from equation 19 of ACC paper
N_temp1=zeros(n,6); N_temp2=zeros(n,6); N_temp3=zeros(n,6);

for i=1:n
    N_temp1=N_temp1+transpose(A_partial(6,n,i).*q_dot_m(i)); % transpose of (6xn times 1x1)
    N_temp2(i,1:6)=transpose(q_dot_m)*transpose(A_partial(6,n,i)); %1xn times nx6
    N_temp3(i,1:6)=0.5*transpose(P)*M0_partial(1:6,1:6,i); % 1x6 times 6x6
end

N_hat=transpose(A)*transpose(adjoint_low(V))*P-N_temp1*P+N_temp2*P+N_temp3*P;

== matlab function Dynamics_v2_temp/Jacobian/MATLAB Function ==
  data: robot input; J output; q input
function J =Jacobian_0(robot,q)
% Compute the geometric Jacobian of the point rp
%   	rp  point of interest in inertial frame 
%       i   link number

% Initiate
J=zeros(6,robot.vehicle.b + robot.n);
% Jm=zeros(6,robot.n);

% Vehicle portion
J0=[robot.vehicle.iota_0];

% ____________ Manipulator Jacobian _____________ %

j=1;
Jm(1:6,j)=robot.joints(j).xi;%[eye(3),zeros(3,3);SkewSym(rL(1:3,j)-rp),eye(3)]*pm(1:6,j);
for j=2:robot.n %Iterate through all joints
    temp=simplify(Adjoint(g(robot.joints(j-1).xi,q(j-1)))*robot.joints(j).xi);%[eye(3),zeros(3,3);SkewSym(rL(1:3,j)-rp),eye(3)]*pm(1:6,j);
    Jm(1:6,j)=temp;
end

Jm=simplify(Jm);

J=[J0 Jm(1:6,1:j)];

end

== matlab function Dynamics_v2_temp/Simulink Function4/MATLAB Function ==
  data: q_m input; q_dot_m input; Xi_m input; M0 input; M0m input; C_hat output; A input; V_I0 input
function C_hat = C_hat(q_m,q_dot_m,Xi_m,M0,M0m,A,V_I0)
% Calculates the C_hat_m matrix from base pose and arm joint angles

n=length(q_m);

% Find the connection A
% [M0, M0m, Mm]=Mass_Matrix(I0,Im,m0,mm,Tij,Ti0,q_m,Xi_m);
% A=inverse(M0)*M0m;

% Find the spaccecraft velocity V
% V=inverse(M0)*(P-transpose(A)*q_dot_m);
V=V_I0;

% Find Lm0
for i=1:n
    Lm0=Ad_frak(1,i,Xi_m,q_m);% equation 63 of TRO
end

% Find partial of Lm0 to joint angles
Lm0_partial=zeros(6*n,6,n); % 6nx6xn
for i=1:n
    for j=1:n
        Lm0_partial(6*(j-1)+1:6*j,1:6,i)=Ad_partial(j,1,i,Xi_m,q_m); % equation 114 of TRO paper
    end
end

% Find partial of M0 to joint angles
M0_partial=zeros(6,6,n); %initiate
for i=1:n
    M0_partial(1:6,1:6,i)= transpose(Lm0_partial(i))*diagM*Lm0+transpose(Lm0)*diagM*Lm0_partial(i); %6x6 %equation 117 of TRO
end

% Find partial of M0m to joint angles
M0m_partial=zeros(6,n,n);
for i=1:n
    M0m_partial(6,n,i)= (transpose(Lm0_partial)*diagM*Lm0+transpose(Lm0)*diagM*Lm)*Xi_m_matrix; % equation 118 of TRO paper
end

% Find partial of connection A to each joint angle
A_partial=zeros(6,n,n);
for i=1:n
    A_partial(6,n,i)=inverse(M0)*M0_partial(1:6,1:6,i)*inverse(M0)*M0m+inverse(M0)*M0m_partial(6,n,i); % Equation 122
end

% find the non-generalized arm mass matrix'x derivative to joint angles
for i=1:n
    Mm_partial(i)=transpose(Xi_m)*(transpose(Lm_partial(i))Lm + ...
        transpose(Lm)*()*Lm_partial(i))*Xi_m; %calcualte the derivative of not-augmented arm mass matrix from equation 120 of TRO paper
end

% find the temp intermediate term
for i=1:n
    AMA_partial(i)=transpose(A_partial(6,n,i))*M0*A+transpose(A)*M0_partial(i)*A+transpose(A)*M0*A_partial(6,n,i); %calcualte the derivative of not-augmented arm mass matrix from equation 121 of TRO paper
end

for i=1:n
    Mm_hat_partial(i)=Mm_partial(i)-AMA_partial(i); %calcualte the derivative of augmented arm mass matrix from equation 119 of TRO paper
end

for i=1:n
    C_temp1=C_temp1+Mm_hat_partial(n,n,i).*q_dot_m(i); % nxn by 1x1
    C_temp2()=0.5*transpose(q_dot_m)*Mm_hat_partial(n); %1xn by nx1 
end

C_hat=C_temp1-C_temp2;

== matlab function Dynamics_v2_temp/Simulink Function2/Mass Matrix Blocks/Mass_Matrix_Blocks1 ==
  data: m_diag input; Lm0 input; Lm input; Xi_m_matrix input; M0 output; M0m output; Mm output; iota0 input
function [M0,M0m,Mm]=Mass_Matrix(m_diag,Lm0,Lm,Xi_m_matrix,iota0)
% Compute the Mass Matrix of the multibody system.
%   Output:
%   M0      Spacecraft mass matrix 
%   M0m
%   Mm      Manipulator mass matrix

%n=length(q_m);

m0_frak=m_diag(1:6,1:6);
m_diag=m_diag(7:end,7:end);

%Initiate
M0=[I0,zeros(3,3);zeros(3,3),m0*eye(3)];
M0m=zeros(6,6*n);
Mm=zeros(6*n,6*n);

%calculate transposes
iota0T=transpose(iota0);
Lm0T=transpose(Lm0);
LmT=transpose(Lm);
Xi_mT=transpose(Xi_m_matrix);

% Vehicle Spacecraft Mass matrix block
M0=iota0T*(m0_frak+Lm0T*m_diag*Lm0)*iota0;

% Vehicle Spacecraft Mass matrix block
M0m=iota0T*Lm0T*m_diag*Lm*Xi_m_matrix;

% Vehicle Spacecraft Mass matrix block
Mm=Xi_mT*LmT*m_diag*Lm*Xi_m_matrix;



end

== matlab function Dynamics_v2_temp/Simulink Function6/MATLAB Function ==
  data: I0 input; Im input; m0 input; mm input; Tij input; Ti0 input; M0 output; q_m input; M0m output; Mm output; Xi_m input
function [M0,M0m,Mm]=Mass_Matrix(I0,Im,m0,mm,Tij,Ti0,q_m,Xi_m)
% Compute the Mass Matrix of the multibody system.
%   Output:
%   M0      Spacecraft mass matrix 
%   Mm      Manipulator mass matrix

n=length(q_m);

%Initiate
Mm=zeros(6,6,n,'like',I0);

% Calculate L matrix
for i=1:n
    for j=1:n
        if i>j
            Ad_temp=eye(6);
            for k=i:j
                Ad_temp=Ad_temp*Adjoint(g_matrix(-Xi_m(k),q_m(k)))
            end
            L(6*(i-1)+1:6*(i-1)+6,6*(j-1)+1:6*(j-1)+6)=Ad_temp;
        elseif i==j
            L(6*(i-1)+1:6*(i-1)+6,6*(j-1)+1:6*(j-1)+6)=zeros(6);
        elseif i<j
            L(6*(i-1)+1:6*(i-1)+6,6*(j-1)+1:6*(j-1)+6)=zeros(6);
        end
    end
end

%Backwards recursion
for i=n:-1:1
    %Initialize M 
    Mm(1:6,1:6,i)=[Im(1:3,1:3,i),zeros(3,3);zeros(3,3),mm(i)*eye(3)];
    for j=1:n-i
        Mm(1:6,1:6,i)=Mm_tilde(1:6,1:6,i)+Tij(1:6,1:6,i+j,i)'*Mm(1:6,1:6,i+j)*Tij(1:6,1:6,i+j,i);
        % Conjugation of the Inertia matrix by the translation matrix corresponding to CG
    end
end

% Spacecraft M tilde
M0=[I0,zeros(3,3);zeros(3,3),m0*eye(3)];
for j=1:n
    M0=M0+Ti0(1:6,1:6,j)'*Mm(1:6,1:6,j)*Ti0(1:6,1:6,j);
end


end

== matlab function Dynamics_v2_temp/Simulink Function5/MATLAB Function ==
  data: M0 input; M0m input; A output
function A=A_connection(M0,M0m)
% Compute the connection A from mass properties

A=M0\M0m;

== matlab function Dynamics_v2_temp/Simulink Function7/MATLAB Function ==
  data: P input; A_connection input; q_dot_m input; M0 input; V_I0 output
function V_I0=V_I0(P,A_connection,q_dot_m,M0)
% Find the spaccecraft velocity V_I0
V_I0=inverse(M0)*(P-transpose(A_connection)*q_dot_m);

== matlab function Dynamics_v2_temp/Simulink Function8/MATLAB Function ==
  data: g_I0 input; mu input; P output
function P=Momentum(g_I0,mu)
% find the momentum in current base frame
P=transpose(Adjoint(g_I0))*mu;

== matlab function Dynamics_v2_temp/Simulink Function9/MATLAB Function ==
  data: M0_partial output; q_m input; M0m_partial output; Mm_partial output; Xi_m input
function [M0_partial,M0m_partial,Mm_partial]=Mass_Derivatives(q_m,Xi_m)
% Compute the Mass Matrix of the multibody system.
%   Output:
%   M0      Spacecraft mass matrix 
%   Mm      Manipulator mass matrix

n=length(q_m);

% Find Lm0
for i=1:n
    Lm0=Ad_frak(1,i,Xi_m,q_m);% equation 63 of TRO
end

% Find partial of Lm0 to joint angles
Lm0_partial=zeros(6*n,6,n); % 6nx6xn
for i=1:n
    for j=1:n
        Lm0_partial(6*(j-1)+1:6*j,1:6,i)=Ad_partial(j,1,i,Xi_m,q_m); % equation 114 of TRO paper
    end
end

% Find partial of M0 to joint angles
M0_partial=zeros(6,6,n); %initiate
for i=1:n
    M0_partial(1:6,1:6,i)= transpose(Lm0_partial(i))*diagM*Lm0+transpose(Lm0)*diagM*Lm0_partial(i); %6x6 %equation 117 of TRO
end

% Find partial of M0m to joint angles
M0m_partial=zeros(6,n,n);
for i=1:n
    M0m_partial(6,n,i)= (transpose(Lm0_partial)*diagM*Lm0+transpose(Lm0)*diagM*Lm)*Xi_m_matrix; % equation 118 of TRO paper
end

% Find partial of connection A to each joint angle
A_partial=zeros(6,n,n);
for i=1:n
    A_partial(6,n,i)=inverse(M0)*M0_partial(1:6,1:6,i)*inverse(M0)*M0m+inverse(M0)*M0m_partial(6,n,i); % Equation 122
end

== matlab function Dynamics_v2_temp/Simulink Function13/  ==
  data: q_m input; L0 output; Lm0 output; Lm output; Xi_m input
function [L0,Lm0,Lm] =L_calculator(q_m,Xi_m)
% Calculates the time-dependent L matrix
n=length(q_m);
L=zeros(6*(n+1),6*(n+1));
% Compute M_frak for ith body
% Calculate L matrix
for i=1:n
    for j=1:n
        if i>j
            Ad_temp=eye(6);
            for k=i:j
                Ad_temp=Ad_temp*Adjoint(g_Matrix(-Xi_m(:,k),q_m(k)));
            end
            L(6*(i-1)+1:6*(i-1)+6,6*(j-1)+1:6*(j-1)+6)=Ad_temp;
        elseif i==j
            L(6*(i-1)+1:6*(i-1)+6,6*(j-1)+1:6*(j-1)+6)=eye(6);
        elseif i<j
            L(6*(i-1)+1:6*(i-1)+6,6*(j-1)+1:6*(j-1)+6)=zeros(6);
        end
    end
end

L0=L(1:6,1:6);
Lm0=L(7:end,1:6);
Lm=L(7:end,7:end);

end

== matlab function Dynamics_v2_temp/Simulink Function2/diag M_frak/Subsystem/M_frak array ==
  data: M_curly0 input; I0 input; M_curlym input; II input; g_bar input; M_frak output
function M_frak =M_frak(M_curly0,I0,M_curlym,II,g_bar)
% Compute M_frak for ith body

for i=1:n
    Ad_g_bar(i,:,:)=Adjoint(g_bar(i,:,:));
    Ad_g_bar_inv(i,:,:)=inv(Ad_g_bar(i,:,:));
end

% Calculate M_hat
for i=1:n
    M_frak(i,:,:)=transpose(Ad_g_bar_inv(i,:,:))*M_curly(i,:,:)*Ad_g_bar(i,:,:);
end

== matlab function Dynamics_v2_temp/Simulink Function2/diag M_frak/MATLAB Function1 ==
  data: M_frak input; diag_M output
function diag_M =diagonalize(M_frak)
% Compute M_frak for ith body
n=length(M_frak(:,1,1));
% Initiate
diag_M=zeros(6*n,6*n);
% Calculate diag{M_frak}
for i=1:6*n
    diag_M(6*(i-1)+1:6*i,6*(i-1)+1:6*i)=M_frak(i,:,:);
end

end

== matlab function Dynamics_v2_temp/Simulink Function15/MATLAB Function ==
  data: m0 input; M_curly output; I0 input; mm input; Im input; g_cm input
function M_curly= M_curly(m0,I0,mm,Im,g_cm)

% form set of M in the joint frames
M_curly0(:,:)=[m0*eye(3,3);zero(3,3);zeros(3,3);I0];
for i=1:n
    M_curly(i,:,:)=[mm(i)*eye(3,3);zero(3,3);zeros(3,3);II(i,:,:)];
end

== matlab function Dynamics_v2_temp/Simulink Function14/MATLAB Function1 ==
  data: A input; A_inv output
function A_inv=Mat_inv(A)
% Computes inverse of a matrix
% singularity not yet implemented

A_inv=inv(A);

end

== matlab function Dynamics_v2_temp/Inverse Dynamics/Euler Poincare/MATLAB Function ==
  data: V input; adj_low output; iota0 input
function adj_low = adj_low(V, iota0)
% calculates the adjoint corresponding to the Lie bracket of vector V and ()
adj_low = adjoint_low(V,iota0);

== matlab function Dynamics_v2_temp/Simulink Function16/MATLAB Function ==
  data: g input; Adj output
function Adj  = Adjoint(g)
% returns the adjoint of the given transformation
    R=zeros(3);     R=g(1:3,1:3);
    p=zeros(3,1);   p=g(1:3,4);
    Adj=[R skewsym(p)*R;zeros(3) R];
endfunction y = fcn(u)

y = u;

== matlab function Dynamics_v2_temp/Simulink Function10/MATLAB Function ==
  data: M0 input; Mm input; A input; M_hat output
function M_hat =M_hat(M0,Mm,A)
% Compute the Mass Matrix of the multibody system.
%   Input:
%   M0      Spacecraft mass matrix 
%   M0m     Coupling
%   Mm      Manipulator mass matrix

% Calculate M_hat
M_hat=Mm-transpose(A)*M0*A;


end

== matlab function Dynamics_v2_temp/Simulink Function15/MATLAB Function1 ==
  data: xi input; qm input; g output
function g  = g_Matrix(xi,qm) %#codegen
% compute the tranformation matrix containing the rotation matrix R and
% the translation vector s between two joints

%Revolute joint
theta=qm;
  
% Form the g Matrix
g=expm(xi*theta)*g_bar;
% g=inv([eye(3),b;zeros(1,3),1])*[R,s;zeros(1,3),1];

end

== matlab function Dynamics_v2_temp/time-dependent variables' calculations/Jacobian End Effector/Forward Kinematics ==
  data: g_0e output; q_m input; Xi_m input; g_bar input
function g_0e = Forward_Kinematics(q_m,Xi_m,g_bar)
% Calculates the absolute pose of end-effector from base pose and arm joint angles

n=length(q_m);

% Initiate
g_bar_ee=eye(4,4); %the initial pose of the end-effector
g_0e=eye(4,4); %the pose of the end-effector

for i=1:n
    g_bar_ee=g_bar_ee*squeeze(g_bar(:,:,i));
end

for i=1:n
%     g_0e=g_0e*expm(skewsym(Xi_m(1:6,i)).*q_m(i)); % the effect of the motion induced by each joint
    g_0e=g_0e*g_Matrix(Xi_m(1:6,i),q_m(i)); % the effect of the motion induced by each joint
end

g_0e=g_0e*g_bar_ee; %multiply by the initial pose of the last link (wrist)

== matlab function Dynamics_v2_temp/Inverse Dynamics/Internal Dynamics/Inverse ==
  data: M_hat input; M_hat_inverse output
function M_hat_inverse = Inverse(M_hat)

M_hat_inverse=inv(M_hat);

== matlab function Dynamics_v2_temp/Inverse Dynamics/Internal Dynamics/C_hat/C_hat ==
  data: q_m input; q_dot_m input; C_hat output; Mm_hat_partial input
function C_hat = C_hat(q_m,q_dot_m, Mm_hat_partial)
% Calculates the C_hat_m matrix from base pose and arm joint angles

n=length(q_m);


% Calculate C_hat matrix
C_temp1=zeros(n,n);
C_temp2=zeros(n,n);
C_hat=zeros(n,n);
for i=1:n
    C_temp1=C_temp1+Mm_hat_partial(1:n,1:n,i).*q_dot_m(i); % nxn by scalar
    C_temp2(i,1:n)=0.5*transpose(q_dot_m)*Mm_hat_partial(1:n,1:n,i); %1xn by nxn 
end

C_hat=C_temp1-C_temp2;

== matlab function Dynamics_v2_temp/Inverse Dynamics/Internal Dynamics/C_hat/Lm_partials/Lm0partial ==
  data: q_m input; Lm0_partial output; Xi_m input; iota0 input
function Lm0_partial = Lm0_partial(q_m,Xi_m,iota0)
% Calculates the C_hat_m matrix from base pose and arm joint angles

n=length(q_m);

% Find partial of Lm to joint angles
Lm0_partial=zeros(6*n,6,n); % 6nx6xn
for i=1:n
    for j=1:n
        Lm0_partial(6*(j-1)+1:6*j,1:6,i)=Ad_partial(j,1,i,Xi_m,q_m,iota0); % equation 114 of TRO paper
    end
end

== matlab function Dynamics_v2_temp/Inverse Dynamics/Internal Dynamics/M_hat ==
  data: M0 input; Mm input; A input; M_hat output
function M_hat =M_hat(M0,Mm,A)
% Compute the Mass Matrix of the multibody system.
%   Input:
%   M0      Spacecraft mass matrix 
%   M0m     Coupling
%   Mm      Manipulator mass matrix

% Calculate M_hat
M_hat=Mm-transpose(A)*M0*A;


end
